simulink model "motor"  (R2021b)
settings: Solver=VariableStepAuto  StartTime=0.0  StopTime=0.15  FixedStep=0.001  RelTol=1e-3
settings Model: Creator=suzer  LastModifiedBy=suzer

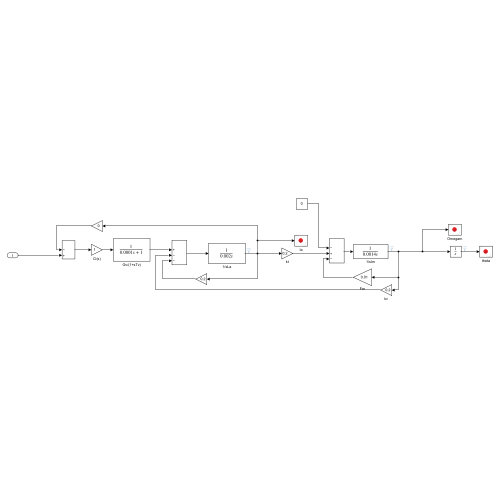
[thumbnail: Simulink's stored preview of the top-level diagram]
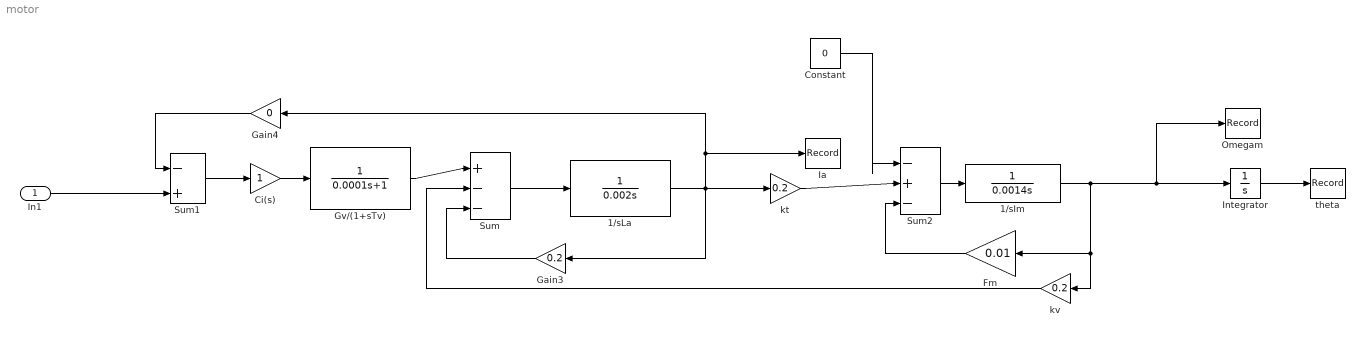
== system motor ==
  In1 : Inport
  1/sIm : TransferFcn  Denominator=[0.0014 0]
  1/sLa : TransferFcn  Denominator=[0.002 0]
  Ci(s) : Gain
  Constant : Constant  Value=0
  Fm : Gain  Gain=0.01
  Gain3 : Gain  Gain=0.2
  Gain4 : Gain  Gain=0
  Gv/(1+sTv) : TransferFcn  Denominator=[0.0001 1]
  Ia : Record  FileSettingsInternal="{\"entries\":[{\"content\":{\"excelSettings\":{\"content\":{},\"type\":\"Streamout.ExcelSettings\"}},\"type\":\"Streamout.FileSettingStorage\",\"uuid\":\"523acee1-ef40-4f74-a76e-5276b4e9ac07\"}],\"packageUris\":[\"http://schema.mathworks.com/mf0/streamout_blocks/R2020a\"],\"version\":\"1.0\"}"  Layout=[1 1]  SignalsInternal="{\"entries\":[{\"content\":{\"signals\":[{\"content\":{\"blockPath\":[\"motor/Ia\"],\"channel\":[],\"dimensions\":[1],\"domain\":\"motor/Ia\",\"lineColor\":\"#ff13a6\",\"plots\":[1],\"port\":1,\"sid\":[],\"signalID\":27,\"signalName\":\"1/sLa\"},\"type\":\"RecordBlkView.Signal\",\"uuid\":\"67ea8a6e-bf76-442c-9edb-bc740b76482a\"}]},\"type\":\"RecordBlkView.InputSignals\",\"uuid\":\"88271dac-3f77-4e5d-82e4-8288721009dd\"}],\"packageUris\":[\"http://schema.mathworks.com/mf0/streamout_blocks/R2020a\"],\"version\":\"1.0\"}"
  Integrator : Integrator
  Omegam : Record  FileSettingsInternal="{\"entries\":[{\"content\":{\"excelSettings\":{\"content\":{},\"type\":\"Streamout.ExcelSettings\"}},\"type\":\"Streamout.FileSettingStorage\",\"uuid\":\"32a12994-518c-421f-bed2-195b6e8a8302\"}],\"packageUris\":[\"http://schema.mathworks.com/mf0/streamout_blocks/R2020a\"],\"version\":\"1.0\"}"  Layout=[1 1]  SignalsInternal="{\"entries\":[{\"content\":{\"signals\":[{\"content\":{\"blockPath\":[\"motor/Omegam\"],\"channel\":[],\"dimensions\":[1],\"domain\":\"motor/Omegam\",\"lineColor\":\"#fe330a\",\"plots\":[1],\"port\":1,\"sid\":[],\"signalID\":22,\"signalName\":\"1/sIm\"},\"type\":\"RecordBlkView.Signal\",\"uuid\":\"2d353e53-b526-475c-b44a-61e7b3973ee7\"}]},\"type\":\"RecordBlkView.InputSignals\",\"uuid\":\"26073e19-b5d8-4666-8d70-9b2ffe5e3834\"}],\"packageUris\":[\"http://schema.mathworks.com/mf0/streamout_blocks/R2020a\"],\"version\":\"1.0\"}"
  Sum : Sum  Inputs=|+--
  Sum1 : Sum  Inputs=|-+
  Sum2 : Sum  Inputs=|-+-
  kt : Gain  Gain=0.2
  kv : Gain  Gain=0.2
  theta : Record  FileSettingsInternal="{\"entries\":[{\"content\":{\"excelSettings\":{\"content\":{},\"type\":\"Streamout.ExcelSettings\"}},\"type\":\"Streamout.FileSettingStorage\",\"uuid\":\"43595d06-c307-4114-940e-04d73374a12b\"}],\"packageUris\":[\"http://schema.mathworks.com/mf0/streamout_blocks/R2020a\"],\"version\":\"1.0\"}"  Layout=[1 1]  SignalsInternal="{\"entries\":[{\"content\":{\"signals\":[{\"content\":{\"blockPath\":[\"motor/theta\"],\"channel\":[],\"dimensions\":[1],\"domain\":\"motor/theta\",\"lineColor\":\"#edb120\",\"plots\":[1],\"port\":1,\"sid\":[],\"signalID\":17,\"signalName\":\"Integrator\"},\"type\":\"RecordBlkView.Signal\",\"uuid\":\"f6256925-441e-4336-aba3-73d79dafa0f0\"}]},\"type\":\"RecordBlkView.InputSignals\",\"uuid\":\"403e547e-ebc3-4cdc-b338-577637b8faae\"}],\"packageUris\":[\"http://schema.mathworks.com/mf0/streamout_blocks/R2020a\"],\"version\":\"1.0\"}"
  wires:
  Constant/1 -> Sum2/1
  Gv/(1+sTv)/1 -> Sum/1
  Sum1/1 -> Ci(s)/1
  Ci(s)/1 -> Gv/(1+sTv)/1
  Sum2/1 -> 1/sIm/1
  kt/1 -> Sum2/2
  Gain4/1 -> Sum1/1
  Sum/1 -> 1/sLa/1
  Fm/1 -> Sum2/3
  kv/1 -> Sum/2
  Integrator/1 -> theta/1
  1/sLa/1 -> Gain4/1, Ia/1, Gain3/1, kt/1
  Gain3/1 -> Sum/3
  1/sIm/1 -> kv/1, Fm/1, Integrator/1, Omegam/1
  In1/1 -> Sum1/2
